simulink model "SimpleSubscriber"  (R2021a)
settings: Solver=VariableStepAuto  StartTime=0.0  StopTime=inf  RelTol=1e-3
libraries: robotlib x1
settings Model: Creator=iris  LastModifiedBy=iris

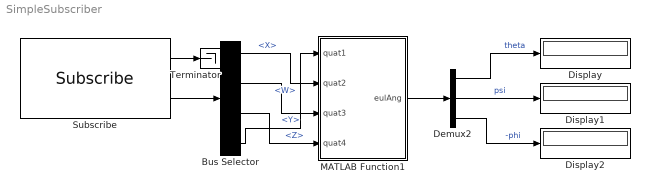
== system SimpleSubscriber ==
  Bus Selector : BusSelector  OutputSignals=Pose.Pose.Orientation.X,Pose.Pose.Orientation.Y,Pose.Pose.Orientation.Z,Pose.Pose.Orientation.W
  Demux2 : Demux  Outputs=3
  Display : Display
  Display1 : Display
  Display2 : Display
  MATLAB Function1 : MATLAB Function  TreatAsAtomicUnit=on
  Subscribe : robotlib/Subscribe  topicSource=Specify your own  topic=/odom  messageType=nav_msgs/Odometry  SampleTime=-1  legacyBusStruct=off  messageQueueLength=1
  Terminator : Terminator
  wires:
  Demux2/2 -> Display1/1  "psi"
  Demux2/3 -> Display2/1  "-phi"
  Subscribe/2 -> Bus Selector/1
  MATLAB Function1/1(eulAng) -> Demux2/1
  Bus Selector/2 -> MATLAB Function1/3(quat3)  "<Y>"
  Subscribe/1 -> Terminator/1
  Bus Selector/1 -> MATLAB Function1/2(quat2)  "<X>"
  Bus Selector/3 -> MATLAB Function1/4(quat4)  "<Z>"
  Bus Selector/4 -> MATLAB Function1/1(quat1)  "<W>"
  Demux2/1 -> Display/1  "theta"

== matlab function SimpleSubscriber/MATLAB Function1 ==
  data: quat1 input; eulAng output; quat2 input; quat3 input; quat4 input
function eulAng = quat2euler(quat1,quat2,quat3,quat4)

quat = [quat1, quat2, quat3, quat4];
eulAng = quat2eul(quat,'ZYX');

end
